simulink model "Calcolator_Sub_sys"  (R2021a)
settings: Solver=FixedStepDiscrete  StartTime=0.0  StopTime=10.0  RelTol=1e-3  EnableMultiTasking=on
settings Model: Creator=alyma  LastModifiedBy=alyma
settings DataIOCC: ReturnWorkspaceOutputs=off
settings OptimizationCC: DefaultParameterBehavior=Inlined  InlineInvariantSignals=on  EnableMemcpy=off  LifeSpan=1  EfficientTunableParamExpr=on
settings DebuggingCC: UnderspecifiedInitializationDetection=Classic  MergeDetectMultiDrivingBlocksExec=none  SFMachineParentedDataDiag=warning  ArithmeticOperatorsInVariantConditions=warning
settings ModelReferenceCC: PropagateSignalLabelsOutOfModel=off
settings SFSimCC: MATLABDynamicMemAlloc=off  CustomCodeUndefinedFunction=UseInterfaceOnly
settings RTWCC: SystemTargetFile=ert.tlc  GenCodeOnly=on  TemplateMakefile=ert_default_tmf  GenerateReport=on  IncludeHyperlinkInReport=on  LaunchReport=on  GenerateTraceInfo=on  GenerateTraceReport=on  GenerateTraceReportSl=on  GenerateTraceReportSf=on  GenerateTraceReportEml=on
settings CodeAppCC: ForceParamTrailComments=on  IgnoreCustomStorageClasses=off  OperatorAnnotations=on  SimulinkDataObjDesc=on  SFDataObjDesc=on  MATLABFcnDesc=on  InsertBlockDesc=on  StateflowObjectComments=on  MATLABSourceComments=on
settings ERTTargetCC: MultiwordLength=2048  GenerateSampleERTMain=on  InlinedParameterPlacement=NonHierarchical  ERTCustomFileTemplate=example_file_process.tlc

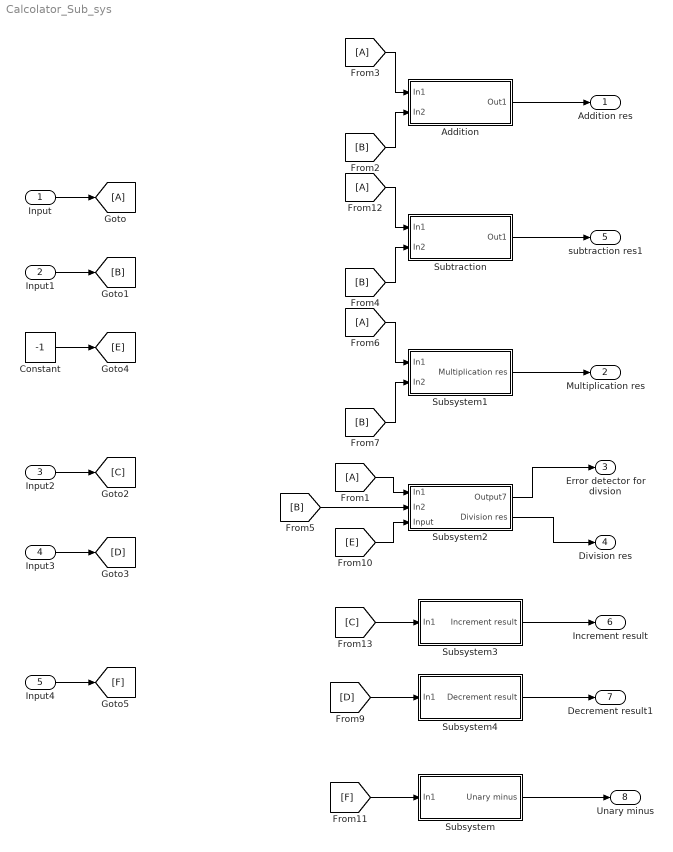
== system Calcolator_Sub_sys ==
  Input : Inport
  Input1 : Inport  Port=2
  Input2 : Inport  Port=3
  Input3 : Inport  Port=4
  Input4 : Inport  Port=5
  Addition : Subsystem
  Constant : Constant  Value=-1
  Subsystem : Subsystem
  Subsystem1 : Subsystem
  Subsystem2 : Subsystem
  Subsystem3 : Subsystem
  Subsystem4 : Subsystem
  "Subtraction " : Subsystem
  Addition res : Outport
  Multiplication res : Outport  Port=2
  Error detector for divsion : Outport  Port=3
  Division res : Outport  Port=4
  subtraction res1 : Outport  Port=5
  Increment result : Outport  Port=6
  Decrement result1 : Outport  Port=7
  Unary minus : Outport  Port=8
  wires:
  Constant/1 -> [E]
  Input1/1 -> [B]
  Input2/1 -> [C]
  Input/1 -> [A]
  Input4/1 -> [F]
  Input3/1 -> [D]
  [A] -> Addition/1(In1)
  [B] -> Addition/2(In2)
  Addition/1(Out1) -> Addition res/1
  [A] -> Subsystem1/1(In1)
  [B] -> Subsystem1/2(In2)
  Subsystem1/1(Multiplication res) -> Multiplication res/1
  Subsystem2/1(Output7) -> Error detector for divsion/1
  [B] -> Subsystem2/2(In2)
  [E] -> Subsystem2/3(Input)
  [A] -> Subsystem2/1(In1)
  Subsystem2/2(Division res) -> Division res/1
  [B] -> "Subtraction "/2(In2)
  [A] -> "Subtraction "/1(In1)
  "Subtraction "/1(Out1) -> subtraction res1/1
  [C] -> Subsystem3/1(In1)
  Subsystem3/1(Increment result) -> Increment result/1
  [D] -> Subsystem4/1(In1)
  Subsystem4/1(Decrement result) -> Decrement result1/1
  Subsystem/1(Unary minus) -> Unary minus/1
  [F] -> Subsystem/1(In1)

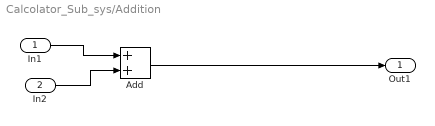
== system Calcolator_Sub_sys/Addition ==
  In1 : Inport
  In2 : Inport  Port=2
  Add : Sum
  Out1 : Outport
  wires:
  Add/1 -> Out1/1
  In2/1 -> Add/2
  In1/1 -> Add/1

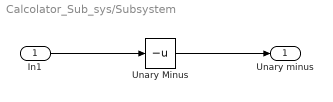
== system Calcolator_Sub_sys/Subsystem ==
  In1 : Inport
  Unary Minus : UnaryMinus
  Unary minus : Outport
  wires:
  In1/1 -> Unary Minus/1
  Unary Minus/1 -> Unary minus/1

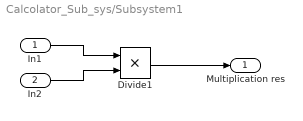
== system Calcolator_Sub_sys/Subsystem1 ==
  In1 : Inport
  In2 : Inport  Port=2
  Divide1 : Product  Inputs=**
  Multiplication res : Outport
  wires:
  Divide1/1 -> Multiplication res/1
  In1/1 -> Divide1/1
  In2/1 -> Divide1/2

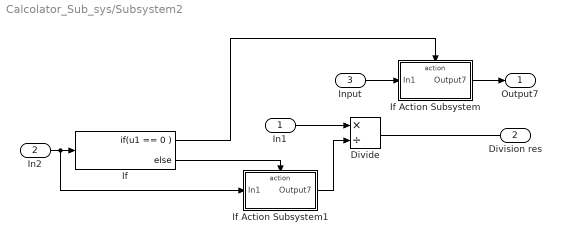
== system Calcolator_Sub_sys/Subsystem2 ==
  In1 : Inport
  In2 : Inport  Port=2
  Input : Inport  Port=3
  Divide : Product  Inputs=*/
  If : If  IfExpression=u1 == 0
  If Action Subsystem : Subsystem  TreatAsAtomicUnit=on
  If Action Subsystem1 : Subsystem  TreatAsAtomicUnit=on
  Output7 : Outport
  Division res : Outport  Port=2
  wires:
  If Action Subsystem1/1(Output7) -> Divide/2
  Input/1 -> If Action Subsystem/1(In1)
  If/2 -> If Action Subsystem1/Action
  In1/1 -> Divide/1
  If/1 -> If Action Subsystem/Action
  In2/1 -> If Action Subsystem1/1(In1), If/1
  Divide/1 -> ?
  If Action Subsystem/1(Output7) -> Output7/1

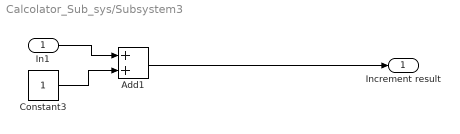
== system Calcolator_Sub_sys/Subsystem3 ==
  In1 : Inport
  Add1 : Sum
  Constant3 : Constant
  Increment result : Outport
  wires:
  In1/1 -> Add1/1
  Add1/1 -> Increment result/1
  Constant3/1 -> Add1/2

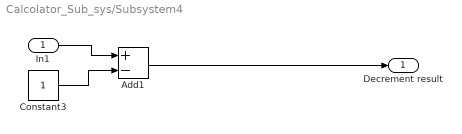
== system Calcolator_Sub_sys/Subsystem4 ==
  In1 : Inport
  Add1 : Sum  Inputs=+-
  Constant3 : Constant
  Decrement result : Outport
  wires:
  In1/1 -> Add1/1
  Add1/1 -> Decrement result/1
  Constant3/1 -> Add1/2

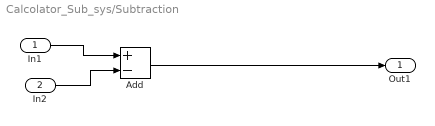
== system Calcolator_Sub_sys/Subtraction  ==
  In1 : Inport
  In2 : Inport  Port=2
  Add : Sum  Inputs=+-
  Out1 : Outport
  wires:
  Add/1 -> Out1/1
  In2/1 -> Add/2
  In1/1 -> Add/1

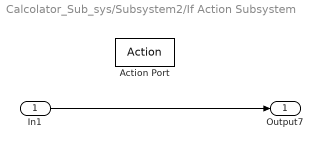
== system Calcolator_Sub_sys/Subsystem2/If Action Subsystem ==
  In1 : Inport
  Action Port : ActionPort  ActionPortLabel=if(u1 == 0 )
  Output7 : Outport
  wires:
  In1/1 -> Output7/1

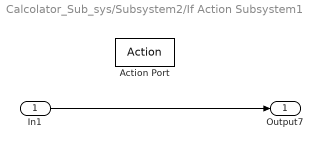
== system Calcolator_Sub_sys/Subsystem2/If Action Subsystem1 ==
  In1 : Inport
  Action Port : ActionPort  ActionPortLabel=else
  Output7 : Outport
  wires:
  In1/1 -> Output7/1
